simulink model "DefaultTransitiontoJunction2"  (R2020b)
settings: Solver=VariableStepAuto  StartTime=0.0  StopTime=10.0  RelTol=1e-3
settings Model: Creator=apple  LastModifiedBy=apple

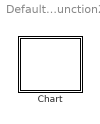
== system DefaultTransitiontoJunction2 ==
  Chart : Stateflow chart  TreatAsAtomicUnit=on

== stateflow chart DefaultTransitiontoJunction2/Chart ==
  state B
    en:fprintf("Entry B");
    du:fprintf("During B");
    ex:fprintf("Exit B");
    state B1
      en:fprintf("Entry B1");
      state B1a
        en:fprintf("Entry B1a");
    state B2
      en:fprintf("Entry B2");
      state B2b
        en:fprintf("Entry B2b");
      state B2a
        en:fprintf("Entry B2a");
      (default) -> B2b
    (default) -> (junction 5)
    (junction 5) -> B2a [order 2]
    (junction 5) -> B1a [order 1] : [x>0]
    B2a -> B1a : [x>-1]
  state A
    en:fprintf("Entry A");
    du:fprintf("During A");
    ex:fprintf("Exit A");
  (default) -> A : {x= 0;}
  A -> B : [x>-5]
  data: x local
